simulink model "ssc_lithium_cell_2RC"  (R2019b)
settings: Solver=ode15s  StartTime=0.0  StopTime=40000  RelTol=1e-3  EnableMultiTasking=on
PreLoadFcn:
  | ssc_lithium_cell_2RC_ini
undefined symbols (not defined in the file): C1_LUT, C2_LUT, Capacity_LUT, cell_Cp_heat, cell_mass, Em_LUT, Qe_init, R0_LUT, R1_LUT, R2_LUT, sigbuilder_block, SOC_LUT, T_init, Temperature_LUT
libraries: fl_lib x11, nesl_utility x6, LiBatteryElements_lib x6, fl_ps_legacy_lib x2
Description:
  | Lithium Battery Cell - Two RC-Branch Equivalent Circuit
  | 
  | This example shows how to model a lithium cell using the Simscape(TM)
  | language to implement the elements of an equivalent circuit model
  | with two RC branches. For the defining equations and their validation,
  | see T. Huria, M. Ceraolo, J. Gazzarri, R. Jackey. "High Fidelity Electrical
  | Model with Thermal Dependence for Characterization and Simulation of
  | High Power Lithium Battery Cells," IEEE International Electric Vehicle
  | Conference, March 2012.
  | 
  | A simple thermal model is used to model battery temperature. It is
  | assumed that cooling is primarily via convection, and that heating is
  | primarily from internal resistance. A battery pack can be modeled by
  | connecting multiple copies of the battery cell block in series.
  | 
  | 
  | 
  | 
  | 
  | 
  | Copyright 2008-2012 The MathWorks, Inc.
settings Model: Creator=MathWorks  LastModifiedBy=bhisma
settings DataIOCC: LimitDataPoints=on  SaveFormat=Array  SignalLoggingSaveFormat=ModelDataLogs  SaveOutput=off  SaveTime=off  ReturnWorkspaceOutputs=off
settings OptimizationCC: ExpressionDepthLimit=2147483647  LifeSpan=inf
settings DebuggingCC: UnderspecifiedInitializationDetection=Classic  MergeDetectMultiDrivingBlocksExec=none  FcnCallInpInsideContextMsg=warning  StateNameClashWarn=warning  SFUnexpectedBacktrackingDiag=warning  SFNoUnconditionalDefaultTransitionDiag=warning  SFExecutionAtInitializationDiag=none  ArithmeticOperatorsInVariantConditions=warning
settings HardwareCC: ProdBitPerPointer=32  ProdBitPerSizeT=32  ProdBitPerPtrDiffT=32  ProdLargestAtomicFloat=None  ProdIntDivRoundTo=Undefined  ProdEndianess=Unspecified  ProdWordSize=32  ProdHWDeviceType=32-bit Generic
settings ModelReferenceCC: PropagateSignalLabelsOutOfModel=off
settings SFSimCC: SimUseLocalCustomCode=off  CustomCodeUndefinedFunction=UseInterfaceOnly
settings RTWCC: RTWUseLocalCustomCode=off
settings CodeAppCC: StateflowObjectComments=on
settings GRTTargetCC: TargetLangStandard=C89/C90 (ANSI)  GeneratePreprocessorConditionals=Disable all  CombineOutputUpdateFcns=off  GRTInterface=on
settings ConfigComp: CovMetricSettings=dw  CovHtmlReporting=on  CovSaveCumulativeToWorkspaceVar=on  CovSaveSingleToWorkspaceVar=on  CovExternalEMLEnable=off
settings SimscapeCC: SimscapeNormalizeSystem=off

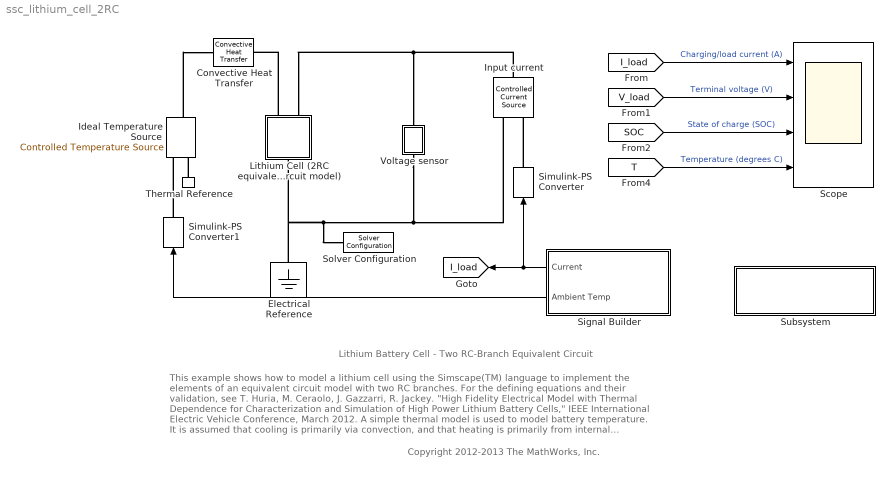
== system ssc_lithium_cell_2RC ==
  note: Lithium Battery Cell - Two RC-Branch Equivalent Circuit
  note: This example shows how to model a lithium cell using the Simscape(TM) language to implement the elements of an equivalent circuit model
      | with two RC branches. For the defining equations and their validation, see T. Huria, M. Ceraolo, J. Gazzarri, R. Jackey. "High Fidelity Electrical
      | Model with Thermal Dependence for Characterization and Simulation of High Power Lithium Battery Cells," IEEE International Electric Vehicle
      | Conference, March 2012. A simple thermal model is used to model battery temperature. It is assumed that cooling is primarily via convection,
      | and that heating is primarily from internal resistance. A battery pack can be modeled by connecting multiple copies of the battery cell block
      | in series.
  note: Copyright 2012-2013 The MathWorks, Inc.
  Convective Heat Transfer : fl_lib/Thermal/Thermal Elements/Convective Heat Transfer  area=cell_area m^2  heat_tr_coeff=h_conv W/(m^2 * K)  T_specify=off  T_priority=None  T=0 K  T_nominal_specify=off  T_nominal_unit=K  T_nominal_value=1  Q_specify=off  Q_priority=None  Q=0 W  Q_nominal_specify=off  Q_nominal_unit=W  Q_nominal_value=1
  Electrical Reference : fl_lib/Electrical/Electrical Elements/Electrical Reference
  Ideal Temperature Source : fl_lib/Thermal/Thermal Sources/Controlled Temperature Source
      settings: SourceProductName=Simscape
  Input current : fl_lib/Electrical/Electrical Sources/Controlled Current Source
  Lithium Cell (2RC equivalent circuit model) : Subsystem  mask(Lithium battery (two RC-branch equivalent circuit)){Qe_init=Qe_init, T_init=T_init, Capacity_LUT=Capacity_LUT, Em_LUT=Em_LUT, R0_LUT=R0_LUT, R1_LUT=R1_LUT, C1_LUT=C1_LUT, R2_LUT=R2_LUT, C2_LUT=C2_LUT, cell_mass=cell_mass, cell_Cp_heat=cell_Cp_heat, SOC_LUT=SOC_LUT, Temperature_LUT=Temperature_LUT}
      mask prompts: Qe_init "Initial charge deficit (A*hr)"; T_init "Initial cell temperature (K)"; Capacity_LUT "Capacity (A*hr, 1xN table)"; Em_LUT "Em open-circuit voltage (volts, MxN table)"; R0_LUT "R0 terminal resistance (ohms, MxN table)"; R1_LUT "R1 resistance (ohms, MxN table)"; C1_LUT "C1 capacitance (farads, MxN table)"; R2_LUT "R2 resistance (ohms, MxN table)"; C2_LUT "C2 capacitance (farads, MxN table)"; cell_mass "Cell mass (kg)"; cell_Cp_heat "Cell specific heat (J/kg/K)"; SOC_LUT "SOC table breakpoints (Mx1 array)"; Temperature_LUT "Temperature table breakpoints(K, 1xN array)"
      mask Display:
      | image(imread('battery.jpg'))
      | color('red')
      | port_label('LConn',1,'H')
      | port_label('LConn',2,'+')
      | port_label('RConn',1,'-')
  Scope : Scope  NumInputPorts=4
  Signal Builder : Subsystem  Tag=STV Subsys  LoadFcn=sigbuilder_block('load');  StartFcn=sigbuilder_block('start');  StopFcn=sigbuilder_block('stop');  ClipboardFcn=sigbuilder_block('clipboard');  mask(Sigbuilder block){tuvar=[0:10]}
      mask help: Simulink:masks:SigbuilderBlock_MD
      mask init:
      | if ~strcmp(get_param(bdroot(gcbh),'SimulationStatus'),'stopped') tuvar = sigbuilder_block('maskInit'); end
      settings: CopyFcn=sigbuilder_block('copy');  DeleteFcn=sigbuilder_block('delete');  ModelCloseFcn=sigbuilder_block('modelClose');  PreSaveFcn=sigbuilder_block('preSave');  PauseFcn=sigbuilder_block('pause');  ContinueFcn=sigbuilder_block('continue');  NameChangeFcn=sigbuilder_block('namechange');  OpenFcn=sigbuilder_block('open',[62.25 82.5 550.5 303 ]);  CloseFcn=sigbuilder_block('close');
      mask Display: plot(0, 0, 100, 100,[2, 2, 32, 32, 2], [68, 8, 8, 68, 68],[32, 2], [38, 38], [32, 19, 2],[53, 60, 44], [32, 17, 17, 2],[16, 16, 31, 31]);txt = getActiveGroup(gcbh);text(2, 100, txt,'verticalAlignment', 'top');
  Simulink-PS Converter : nesl_utility/Simulink-PS Converter  PhysicalDomain=network_engine_domain  SubClassName=ps_input  LeftPortType=input  RightPortType=output  PseudoPeriodic=off  Frequencies=[]  NoiseDistribution=none  NoiseParameters=[]  Unit=A  AffineConversion=off  FilteringAndDerivatives=zero  SimscapeFilterOrder=1  InputFilterTimeConstant=.001  UdotUserProvided=1
  Simulink-PS Converter1 : nesl_utility/Simulink-PS Converter  PhysicalDomain=network_engine_domain  SubClassName=ps_input  LeftPortType=input  RightPortType=output  PseudoPeriodic=off  Frequencies=[]  NoiseDistribution=none  NoiseParameters=[]  Unit=C  AffineConversion=on  FilteringAndDerivatives=zero  SimscapeFilterOrder=1  InputFilterTimeConstant=.001  UdotUserProvided=1
  Solver Configuration : nesl_utility/Solver Configuration  PhysicalDomain=network_engine_domain  SubClassName=solver  LeftPortType=input  RightPortType=generic  Tones=[]  Harmonics=[]  SimulateNoise=off  Profile=off  UseLocalSampling=off  EnableSwitchedLinearOptims=on  FrequencyDomain=off  UseCCode=off  RelTol=0.001  AbsTol=1e-06  MinStep=1e-09  ToWorkspace=off  RevertToSquareIcSolve=off  NumHomotopyIterations=100  PhasorMode=off  PhasorModeNumHarmonics=1  DoDC=off  ResidualTolerance=1e-9  UseLocalSolver=off  LocalSolverChoice=NE_BACKWARD_EULER_ADVANCER  LocalSolverSampleTime=1  DoFixedCost=off  MaxNonlinIter=3  MaxModeIter=2  LinearAlgebra=Sparse  EquationFormulation=NE_TIME_EF  DelaysMemoryBudget=1024  AutomaticFiltering=on  FilteringTimeConstant=0.001  PartitionStorageMethod=AS_NEEDED  PartitionMemoryBudget=1024  PartitionMethod=FAST
  Subsystem : Subsystem
      settings: OpenFcn=open('LiBatteryElements_lib.mdl')
      mask Display: disp('Open the custom\n library used by the\n Lithium Cell block')
  Thermal Reference : fl_lib/Thermal/Thermal Elements/Thermal Reference
  Voltage sensor : Subsystem
  tag scope: I_load=global
  wires:
  [SOC] -> Scope/3  "State of charge (SOC)"
  [T] -> Scope/4  "Temperature (degrees C)"
  [I_load] -> Scope/1  "Charging/load current (A)"
  [V_load] -> Scope/2  "Terminal voltage (V)"
  Signal Builder/2(Ambient Temp) -> Simulink-PS Converter1/1
  Signal Builder/1(Current) -> [I_load], Simulink-PS Converter/1
  connections:
  Electrical Reference/LConn1 -- Lithium Cell (2RC equivalent circuit model)/RConn1 -- Solver Configuration/RConn1 -- Input current/RConn2 -- Voltage sensor/RConn1
  Input current/LConn1 -- Lithium Cell (2RC equivalent circuit model)/LConn2 -- Voltage sensor/LConn1
  Thermal Reference/LConn1 -- Ideal Temperature Source/RConn2
  Ideal Temperature Source/LConn1 -- Convective Heat Transfer/LConn1
  Lithium Cell (2RC equivalent circuit model)/LConn1 -- Convective Heat Transfer/RConn1
  Simulink-PS Converter/RConn1 -- Input current/RConn1
  Simulink-PS Converter1/RConn1 -- Ideal Temperature Source/RConn1

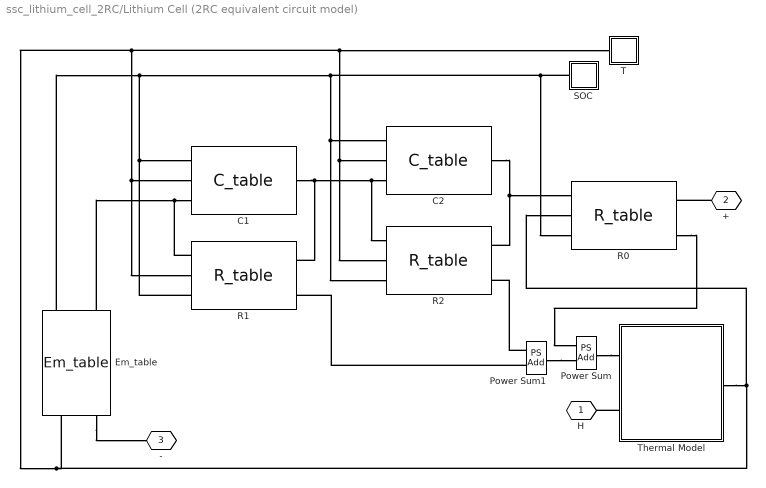
== system ssc_lithium_cell_2RC/Lithium Cell (2RC equivalent circuit model) ==
  " SOC " : Subsystem
  C1 : LiBatteryElements_lib/C_table  C_Table=C1_LUT F  SOC_Table=SOC_LUT  Temp_Table=Temperature_LUT K  v0=0 V
      settings: InternalSimscapePortConfiguration="{\"Bottom\":[],\"Left\":[{\"id\":\"p\",\"label\":\"+\",\"type\":\"foundation.electrical.electrical\"},{\"id\":\"T\",\"label\":\"T\",\"type\":\"input\"},{\"id\":\"SOC\",\"label\":\"SOC\",\"type\":\"input\"}],\"Right\":[{\"id\":\"n\",\"label\":\"-\",\"type\":\"foundation.electrical.electrical\"}],\"Top\":[]}"
  C2 : LiBatteryElements_lib/C_table  C_Table=C2_LUT F  SOC_Table=SOC_LUT  Temp_Table=Temperature_LUT K  v0=0 V
      settings: InternalSimscapePortConfiguration="{\"Bottom\":[],\"Left\":[{\"id\":\"p\",\"label\":\"+\",\"type\":\"foundation.electrical.electrical\"},{\"id\":\"T\",\"label\":\"T\",\"type\":\"input\"},{\"id\":\"SOC\",\"label\":\"SOC\",\"type\":\"input\"}],\"Right\":[{\"id\":\"n\",\"label\":\"-\",\"type\":\"foundation.electrical.electrical\"}],\"Top\":[]}"
  Em_table : LiBatteryElements_lib/Em_table  C_Table=Capacity_LUT hr*A  Em_Table=Em_LUT V  SOC_Table=SOC_LUT  Temp_Table=Temperature_LUT K  Qinit=Qe_init hr*A
      settings: InternalSimscapePortConfiguration="{\"Bottom\":[],\"Left\":[{\"id\":\"p\",\"label\":\"+\",\"type\":\"foundation.electrical.electrical\"},{\"id\":\"C\",\"label\":\"C\",\"type\":\"output\"},{\"id\":\"SOC\",\"label\":\"SOC\",\"type\":\"output\"}],\"Right\":[{\"id\":\"n\",\"label\":\"-\",\"type\":\"foundation.electrical.electrical\"},{\"id\":\"T\",\"label\":\"T\",\"type\":\"input\"}],\"Top\":[]}"
  Power Sum : fl_ps_legacy_lib/Legacy Physical Signals/Functions/PS Add
      settings: SourceProductName=Simscape  SourceProductBaseCode=SS  InternalSimscapePortConfiguration="{\"Bottom\":[],\"Left\":[{\"id\":\"I1\",\"label\":\"\",\"type\":\"input\"},{\"id\":\"I2\",\"label\":\"\",\"type\":\"input\"}],\"Right\":[{\"id\":\"O\",\"label\":\"\",\"type\":\"output\"}],\"Top\":[]}"
  Power Sum1 : fl_ps_legacy_lib/Legacy Physical Signals/Functions/PS Add
      settings: SourceProductName=Simscape  SourceProductBaseCode=SS  InternalSimscapePortConfiguration="{\"Bottom\":[],\"Left\":[{\"id\":\"I1\",\"label\":\"\",\"type\":\"input\"},{\"id\":\"I2\",\"label\":\"\",\"type\":\"input\"}],\"Right\":[{\"id\":\"O\",\"label\":\"\",\"type\":\"output\"}],\"Top\":[]}"
  R0 : LiBatteryElements_lib/R_table  R_Table=R0_LUT Ohm  SOC_Table=SOC_LUT  Temp_Table=Temperature_LUT K
      settings: InternalSimscapePortConfiguration="{\"Bottom\":[],\"Left\":[{\"id\":\"p\",\"label\":\"+\",\"type\":\"foundation.electrical.electrical\"},{\"id\":\"T\",\"label\":\"T\",\"type\":\"input\"},{\"id\":\"SOC\",\"label\":\"SOC\",\"type\":\"input\"}],\"Right\":[{\"id\":\"n\",\"label\":\"-\",\"type\":\"foundation.electrical.electrical\"},{\"id\":\"pow\",\"label\":\"POW\",\"type\":\"output\"}],\"Top\":[]}"
  R1 : LiBatteryElements_lib/R_table  R_Table=R1_LUT Ohm  SOC_Table=SOC_LUT  Temp_Table=Temperature_LUT K
      settings: InternalSimscapePortConfiguration="{\"Bottom\":[],\"Left\":[{\"id\":\"p\",\"label\":\"+\",\"type\":\"foundation.electrical.electrical\"},{\"id\":\"T\",\"label\":\"T\",\"type\":\"input\"},{\"id\":\"SOC\",\"label\":\"SOC\",\"type\":\"input\"}],\"Right\":[{\"id\":\"n\",\"label\":\"-\",\"type\":\"foundation.electrical.electrical\"},{\"id\":\"pow\",\"label\":\"POW\",\"type\":\"output\"}],\"Top\":[]}"
  R2 : LiBatteryElements_lib/R_table  R_Table=R2_LUT Ohm  SOC_Table=SOC_LUT  Temp_Table=Temperature_LUT K
      settings: InternalSimscapePortConfiguration="{\"Bottom\":[],\"Left\":[{\"id\":\"p\",\"label\":\"+\",\"type\":\"foundation.electrical.electrical\"},{\"id\":\"T\",\"label\":\"T\",\"type\":\"input\"},{\"id\":\"SOC\",\"label\":\"SOC\",\"type\":\"input\"}],\"Right\":[{\"id\":\"n\",\"label\":\"-\",\"type\":\"foundation.electrical.electrical\"},{\"id\":\"pow\",\"label\":\"POW\",\"type\":\"output\"}],\"Top\":[]}"
  T : Subsystem
  Thermal Model : Subsystem
  H : PMIOPort  Tag=PMCPort  Side=Left
  + : PMIOPort  Tag=PMCPort  Port=2  Side=Left
  - : PMIOPort  Tag=PMCPort  Port=3  Side=Right
  connections:
  Thermal Model/LConn2 -- H/RConn1
  Em_table/RConn1 -- -/RConn1
  +/RConn1 -- R0/RConn1
  Em_table/LConn1 -- R1/LConn1 -- C1/LConn1
  T/LConn1 -- Thermal Model/RConn1 -- R0/LConn2 -- Em_table/RConn2 -- C1/LConn2 -- R1/LConn2 -- C2/LConn2 -- R2/LConn2
  Power Sum/RConn1 -- Thermal Model/LConn1
  R1/RConn1 -- R2/LConn1 -- C2/LConn1 -- C1/RConn1
  R0/RConn2 -- Power Sum/LConn1
  Power Sum1/RConn1 -- Power Sum/LConn2
  C2/RConn1 -- R0/LConn1 -- R2/RConn1
  Power Sum1/LConn1 -- R2/RConn2
  R1/LConn3 -- C1/LConn3 -- " SOC "/LConn1 -- R0/LConn3 -- C2/LConn3 -- R2/LConn3 -- Em_table/LConn3
  Power Sum1/LConn2 -- R1/RConn2

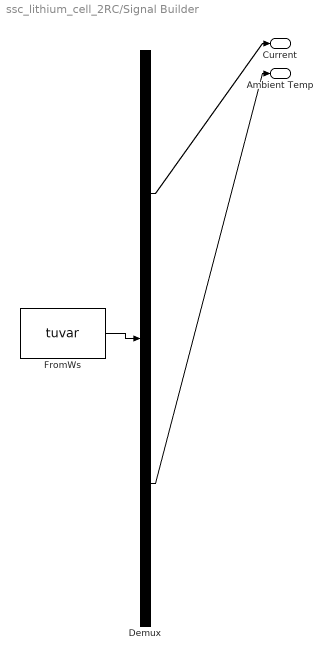
== system ssc_lithium_cell_2RC/Signal Builder ==
  Demux : Demux  Tag=STV Demux  Outputs=2
  FromWs : FromWorkspace  Tag=STV FromWs  VariableName=tuvar  SampleTime=0
      SigBuilderData=|
      | common.afterFinalStr = 'Extrapolate'
      | common.sampleTime = 0
      | dataSet(1).timeRange = [0 40000]
      | dataSet(1).name = 'Pulse'
      | dataSet(2).timeRange = [0 40000]
      | dataSet(2).name = 'Constant'
      | sbobj.Name = 'Signal Builder'
      | sbobj.Groups(1).Name = 'Pulse'
      | sbobj.Groups(1).Signals(1).Name = 'Current'
      | sbobj.Groups(1).Signals(1).XData = [0 300 300 1215 1215 3600 3600 3960 3960 7200 7200 7560 7560 10800 10800 11160 11160 14400 14400 14760 14760 18000 18000 18360 18360 21600 21600 21960 21960 25200 25200 25560 25560 28800 28800 29160 29160 32400 32400 32760 32760 36000 36000 36360 36360 40000]
      | sbobj.Groups(1).Signals(1).YData = [0 0 3.15 3.15 0 0 -4.18 -4.18 0 0 -4.18 -4.18 0 0 -4.18 -4.18 0 0 -4.18 -4.18 0 0 -4.18 -4.18 0 0 -4.18 -4.18 0 0 -4.18 -4.18 0 0 -4.18 -4.18 0 0 -4.18 -4.18 0 0 -4.18 -4.18 0 0]
      | sbobj.Groups(1).Signals(2).Name = 'Ambient Temp'
      | sbobj.Groups(1).Signals(2).XData = [0 300 300 1215 1215 3600 3600 3960 3960 7200 7200 7560 7560 10800 10800 11160 11160 14400 14400 14760 14760 18000 18000 18360 18360 21600 21600 21960 21960 25200 25200 25560 25560 28800 28800 29160 29160 32400 32400 32760 32760 36000 36000 36360 36360 40000]
      | sbobj.Groups(1).Signals(2).YData = [20 20 20 20 20 20 20 20 20 20 20 20 20 20 20 20 20 20 20 20 20 20 20 20 20 20 20 20 20 20 20 20 20 20 20 20 20 20 20 20 20 20 20 20 20 20]
      | sbobj.Groups(1).TimeRange = [0 40000]
      | sbobj.Groups(2).Name = 'Constant'
      | sbobj.Groups(2).Signals(1).Name = 'Current'
      | sbobj.Groups(2).Signals(1).XData = [0 360 360 12500 12500 15800 15800 26500 34500 40000]
      | sbobj.Groups(2).Signals(1).YData = [0 0 -1 -1 0 0 1 1 0 0]
      | sbobj.Groups(2).Signals(2).Name = 'Ambient Temp'
      | sbobj.Groups(2).Signals(2).XData = [0 360 360 12500 12500 15800 15800 26500 34500 40000]
      | sbobj.Groups(2).Signals(2).YData = [20 20.09 20.09 23.125 23.125 23.95 23.95 26.625 28.625 30]
      | sbobj.Groups(2).TimeRange = [0 40000]
  Current : Outport
  Ambient Temp : Outport  Tag=STV Outport  Port=2
  wires:
  FromWs/1 -> Demux/1
  Demux/1 -> Current/1
  Demux/2 -> Ambient Temp/1

== system ssc_lithium_cell_2RC/Subsystem ==

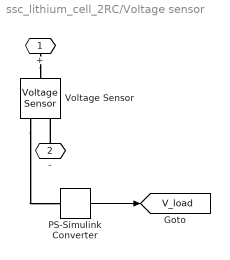
== system ssc_lithium_cell_2RC/Voltage sensor ==
  PS-Simulink Converter : nesl_utility/PS-Simulink Converter  PhysicalDomain=network_engine_domain  SubClassName=ps_output  LeftPortType=input  RightPortType=output  PseudoPeriodic=off  Frequencies=[]  Unit=V  AffineConversion=off
  Voltage Sensor : fl_lib/Electrical/Electrical Sensors/Voltage Sensor
  + : PMIOPort  Side=Left
  - : PMIOPort  Port=2  Side=Right
  tag scope: V_load=global
  wires:
  PS-Simulink Converter/1 -> [V_load]
  connections:
  Voltage Sensor/RConn1 -- PS-Simulink Converter/LConn1
  +/RConn1 -- Voltage Sensor/LConn1
  -/RConn1 -- Voltage Sensor/RConn2

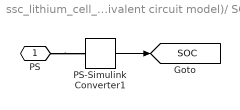
== system ssc_lithium_cell_2RC/Lithium Cell (2RC equivalent circuit model)/ SOC  ==
  PS-Simulink Converter1 : nesl_utility/PS-Simulink Converter  PhysicalDomain=network_engine_domain  SubClassName=ps_output  LeftPortType=input  RightPortType=output  PseudoPeriodic=off  Frequencies=[]  Unit=1  AffineConversion=off
  PS : PMIOPort  Side=Left
  tag scope: SOC=global
  wires:
  PS-Simulink Converter1/1 -> [SOC]
  connections:
  PS/RConn1 -- PS-Simulink Converter1/LConn1

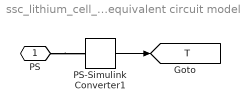
== system ssc_lithium_cell_2RC/Lithium Cell (2RC equivalent circuit model)/T ==
  PS-Simulink Converter1 : nesl_utility/PS-Simulink Converter  PhysicalDomain=network_engine_domain  SubClassName=ps_output  LeftPortType=input  RightPortType=output  PseudoPeriodic=off  Frequencies=[]  Unit=C  AffineConversion=on
  PS : PMIOPort  Side=Left
  tag scope: T=global
  wires:
  PS-Simulink Converter1/1 -> [T]
  connections:
  PS/RConn1 -- PS-Simulink Converter1/LConn1

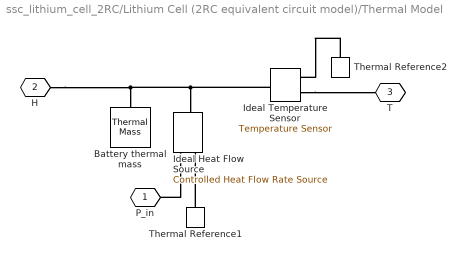
== system ssc_lithium_cell_2RC/Lithium Cell (2RC equivalent circuit model)/Thermal Model ==
  Battery thermal mass : fl_lib/Thermal/Thermal Elements/Thermal Mass  mass=cell_mass kg  sp_heat=cell_Cp_heat J/kg/K  T_specify=on  T_priority=High  T=T_init K  T_nominal_specify=off  T_nominal_unit=K  T_nominal_value=1  Q_specify=off  Q_priority=None  Q=0 W  Q_nominal_specify=off  Q_nominal_unit=W  Q_nominal_value=1
  Ideal Temperature Sensor : fl_lib/Thermal/Thermal Sensors/Temperature Sensor
  Ideal Heat Flow Source : fl_lib/Thermal/Thermal Sources/Controlled Heat Flow Rate Source
      settings: SourceProductName=Simscape
  Thermal Reference1 : fl_lib/Thermal/Thermal Elements/Thermal Reference
  Thermal Reference2 : fl_lib/Thermal/Thermal Elements/Thermal Reference
  P_in : PMIOPort  Tag=PMCPort  Side=Left
  H : PMIOPort  Tag=PMCPort  Port=2  Side=Left
  T : PMIOPort  Tag=PMCPort  Port=3  Side=Right
  connections:
  Thermal Reference2/LConn1 -- Ideal Temperature Sensor/RConn1
  Ideal Temperature Sensor/RConn2 -- T/RConn1
  Thermal Reference1/LConn1 -- Ideal Heat Flow Source/RConn2
  Ideal Temperature Sensor/LConn1 -- H/RConn1 -- Battery thermal mass/LConn1 -- Ideal Heat Flow Source/LConn1
  Ideal Heat Flow Source/RConn1 -- P_in/RConn1
